simulink model "HDVPSG_DelayComp_NewRef_RealDrop_case1"  (R2019b)
settings: Solver=FixedStepDiscrete  StartTime=0.0  StopTime=28  FixedStep=UT.Ts_Veh  RelTol=1e-3
PostLoadFcn:
  | if any(exist('dsrtsu_mdlpostloadfcn', 'file') ~= 0), dsrtsu_mdlpostloadfcn('Execute', bdroot); end
InitFcn:
  | , if any(exist('dsmpb_private', 'file') ~= 0), dsmpb_private('dsmpb_mdlclblib', 'Init', bdroot); end,
values from neighbouring files (symbols this model uses):
  BETA_HDV_Leader = 50    [HDVPSG_DelayComp_NewRef_RealDrop_script_case1.m]
  BETA_PSG_Follower = 150    [HDVPSG_DelayComp_NewRef_RealDrop_script_case1.m]
  CtrlZone_Length = 250    [HDVPSG_DelayComp_NewRef_RealDrop_script_case1.m]
  DELTA_D_MIN = 5    [HDVPSG_DelayComp_NewRef_RealDrop_script_case1.m]
  DELTA_DR_MG_TCC = 15    [HDVPSG_DelayComp_NewRef_RealDrop_script_case1.m]
  HDV_AMAX = 1.3    [HDVPSG_DelayComp_NewRef_RealDrop_script_case1.m]
  HDV_AMIN = -2.5    [HDVPSG_DelayComp_NewRef_RealDrop_script_case1.m]
  HDV_first_v0 = 13    [HDVPSG_DelayComp_NewRef_RealDrop_script_case1.m]
  HDV_HighMu_D = 9    [HDVPSG_DelayComp_NewRef_RealDrop_script_case1.m]
  HDV_HighMu_I = 27    [HDVPSG_DelayComp_NewRef_RealDrop_script_case1.m]
  HDV_HighMu_P = 27    [HDVPSG_DelayComp_NewRef_RealDrop_script_case1.m]
  HDV_HighMu_TRFC = 0.7    [HDVPSG_DelayComp_NewRef_RealDrop_script_case1.m]
  HDV_last_v0 = 13    [HDVPSG_DelayComp_NewRef_RealDrop_script_case1.m]
  HDV_LowMu_D = 6    [HDVPSG_DelayComp_NewRef_RealDrop_script_case1.m]
  HDV_LowMu_I = 8    [HDVPSG_DelayComp_NewRef_RealDrop_script_case1.m]
  HDV_LowMu_P = 12    [HDVPSG_DelayComp_NewRef_RealDrop_script_case1.m]
  HDV_LowMu_TRFC = 0.6    [HDVPSG_DelayComp_NewRef_RealDrop_script_case1.m]
  Np_MPC = 20    [HDVPSG_DelayComp_NewRef_RealDrop_script_case1.m]
  PSG_AMAX = 3.2    [HDVPSG_DelayComp_NewRef_RealDrop_script_case1.m]
  PSG_AMIN = -6    [HDVPSG_DelayComp_NewRef_RealDrop_script_case1.m]
  PSG_end_v0 = 13    [HDVPSG_DelayComp_NewRef_RealDrop_script_case1.m]
  PSG_first_v0 = 13    [HDVPSG_DelayComp_NewRef_RealDrop_script_case1.m]
  PSG_HighMu_D = 15    [HDVPSG_DelayComp_NewRef_RealDrop_script_case1.m]
  PSG_HighMu_I = 125    [HDVPSG_DelayComp_NewRef_RealDrop_script_case1.m]
  PSG_HighMu_P = 75    [HDVPSG_DelayComp_NewRef_RealDrop_script_case1.m]
  PSG_HighMu_TRFC = 0.8    [HDVPSG_DelayComp_NewRef_RealDrop_script_case1.m]
  PSG_LowMu_D = 12    [HDVPSG_DelayComp_NewRef_RealDrop_script_case1.m]
  PSG_LowMu_I = 64    [HDVPSG_DelayComp_NewRef_RealDrop_script_case1.m]
  PSG_LowMu_P = 48    [HDVPSG_DelayComp_NewRef_RealDrop_script_case1.m]
  PSG_LowMu_TRFC = 0.7    [HDVPSG_DelayComp_NewRef_RealDrop_script_case1.m]
  PSG_middle_v0 = 13    [HDVPSG_DelayComp_NewRef_RealDrop_script_case1.m]
  Q_Leader = 1    [HDVPSG_DelayComp_NewRef_RealDrop_script_case1.m]
  Qd_dot_PSG_Follower = 2    [HDVPSG_DelayComp_NewRef_RealDrop_script_case1.m]
  Qd_PSG_Follower = 10    [HDVPSG_DelayComp_NewRef_RealDrop_script_case1.m]
  R_Leader = 20    [HDVPSG_DelayComp_NewRef_RealDrop_script_case1.m]
  R_PSG_Follower = 1    [HDVPSG_DelayComp_NewRef_RealDrop_script_case1.m]
  Recved_40_1 = Recved_Flag_Combined(47740,:)    [HDVPSG_DelayComp_NewRef_RealDrop_script_case1.m]
  Recved_40_2 = Recved_Flag_Combined(47780,:)    [HDVPSG_DelayComp_NewRef_RealDrop_script_case1.m]
  Recved_40_3 = Recved_Flag_Combined(49536,:)    [HDVPSG_DelayComp_NewRef_RealDrop_script_case1.m]
  Recved_40_4 = Recved_Flag_Combined(118106,:)    [HDVPSG_DelayComp_NewRef_RealDrop_script_case1.m]
  Rho_deltad_PSG_Follower = 1e3    (= 1000)    [HDVPSG_DelayComp_NewRef_RealDrop_script_case1.m]
  Rho_v_PSG_Follower = 1e3    (= 1000)    [HDVPSG_DelayComp_NewRef_RealDrop_script_case1.m]
  T_ADE = 0.01    [HDVPSG_DelayComp_NewRef_RealDrop_script_case1.m]
  V_MAX = 40    [HDVPSG_DelayComp_NewRef_RealDrop_script_case1.m]
  V_MIN = 0    [HDVPSG_DelayComp_NewRef_RealDrop_script_case1.m]
  VR_MG_TCC = 15    [HDVPSG_DelayComp_NewRef_RealDrop_script_case1.m]
undefined symbols (not defined in the file or in its folder): DiscIntNeverNeededParam, UT
libraries: simulink x46
(part 1 of 16)
PreSaveFcn:
  | , if any(exist('dsmpb_private', 'file') ~= 0), dsmpb_private('dsmpb_mdlclblib', 'PreSave', bdroot); end,
CloseFcn:
  | , if any(exist('dsmpb_private', 'file') ~= 0), dsmpb_private('dsmpb_mdlclblib', 'Close', bdroot); end,
settings Model: RTICANMMDATA=struct('GeneralSetupData',struct('modelroot',['C:\Program Files (x86)\Eclipse\Sumo\tools\contributed\traci4matlab\ZJ_Learn_Matlab4Traci\CVXGEN_ACM\acm-main\ACM_SUMO_ZJ\Simulink_With_Veh_Dynamics'],'generalsettings',struct('filesettings',struct('destfolder',struct('Name','RTICANMM_FILES','Check',1),'buildfolder',struct('Name','.','Check',1),'AbsDestfolder',struct('Name',['C:\Program Files (x86)\Eclipse\Sumo\tools\contributed\traci4matlab\ZJ_Learn_Matlab4Traci\CVXGEN_ACM\acm-main\ACM_SUMO_ZJ\Simulink_With_Veh_Dynamics\RTICANMM_FILES']),'AbsBuildfolder',struct('Name',['C:\Program Files (x86)\Eclipse\Sumo\tools\contributed\traci4matlab\ZJ_Learn_Matlab4Traci\CVXGEN_ACM\acm-main\ACM_SUMO_ZJ\Simulink_With_Veh_Dynamics']))),'options',struct('addpaths',1,'rmpaths',1,'addtrcexclusion',true,'cannavigator',struct('checkmonitoring',0),'show_usrtrc',0,'use_usrtrc',0),'advanced',struct('options',ones(1,100)),'MPSetup',{{}},'RTI',struct('Type','DSRT','Ver','4.2','Date','02-Nov-2019'),'modelname','HDVPSG_DelayComp_NewRef_RealDrop_case1','block','HDVPSG_DelayComp_NewRef_RealDrop_case1'))  DSRTSU_INTERNAL_RTIFPGA=150  Creator=znq  LastModifiedBy=znq
settings OptimizationCC: BlockReduction=off  ConditionallyExecuteInputs=off  OptimizeBlockIOStorage=off  BufferReuse=off  GlobalBufferReuse=off  ExpressionFolding=off  LocalBlockOutputs=off  OptimizeDataStoreBuffers=off  BusAssignmentInplaceUpdate=off
settings DebuggingCC: TasksWithSamePriorityMsg=none
settings HardwareCC: ProdBitPerPointer=32  ProdBitPerSizeT=32  ProdBitPerPtrDiffT=32  ProdLargestAtomicInteger=Integer  ProdWordSize=32  ProdHWDeviceType=Custom Processor->Custom
settings SFSimCC: MATLABDynamicMemAlloc=off
settings RTWCC: Description=dSPACE Run-Time Target (for VEOS on Windows and ConfigurationDesk)  SystemTargetFile=dsrt.tlc  GenCodeOnly=on  MakeCommand=make_dsrt  TemplateMakefile=dsrt_default_tmf  RTWVerbose=off
settings STFCustomTargetCC: TargetLangStandard=C99 (ISO)  ParMdlRefBuildCompliant=on  SystemTargetFile=dsrt.tlc
settings GRTTargetCC: CompOptLevelCompliant=off  ConcurrentExecutionCompliant=off  CombineOutputUpdateFcns=off  MatFileLogging=off  CPPClassGenCompliant=off  UseToolchainInfoCompliant=off

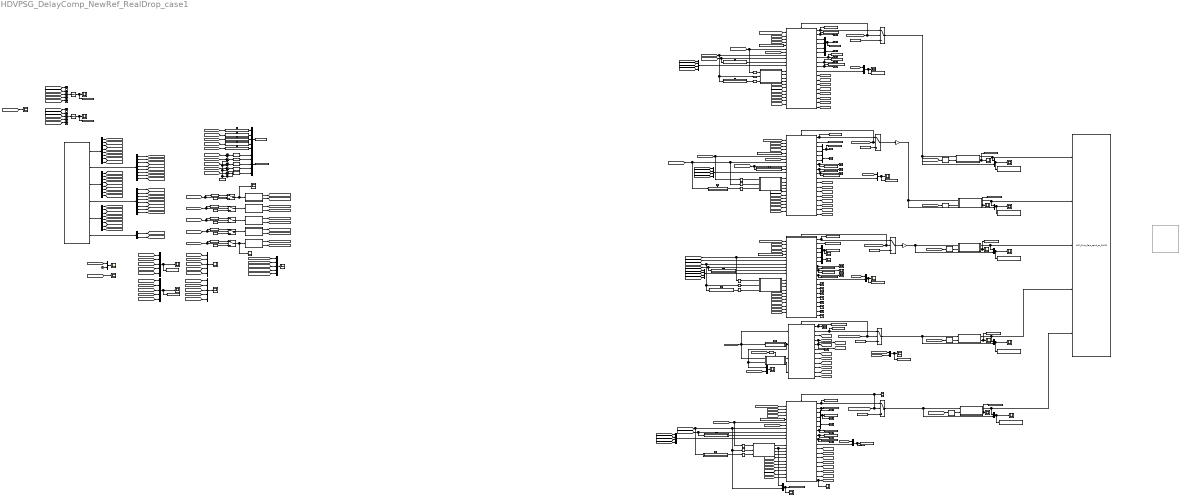
== system HDVPSG_DelayComp_NewRef_RealDrop_case1 ==
  note: We have reset the initial condition, such that FIFO is nautally set.
      | When PSG1 enters, it already has HDV2 inside the CTZ
      | You just say FIFO adopted, others refer to xxxx
  note: Here, we assume the a, v, d of a front car is send from that car, so, for instance, we do not need to calculate the a from its v, by ADE. If not, the control performance may be worsen.
  note: Vehicles Move Inside the Control Zone
  note: For all the merging participant, we assume their PDR are the same
      |
      | However, we cannot assume the package drops occur simutaneously between any two cars
      |
      | So, do not use the same Random Number generator seed
      |
      | Also, we assume the V2V package update rate for all the vehicles are the same
      |
      | Note the V2V package update rate != control rate = 0.01s
      |
      | V2V update slow, then a package drop will result in a longer unchanged V2V message (delay)
      |
      | A more realistic communication simulation may be done with NS3 (Omnet++)
  note: Comparison:
      | Opt / Opt + ULMPC
      | W/O self-prediction
      |
      | Other Seq / Other references refer to IV
      | XY Collision not needed anymore, as the new MP avoids lateral collsion
  ARE_First_Order_Derivative_[1,0,0]1 : Subsystem  TreatAsAtomicUnit=on
  ARE_First_Order_Derivative_[1,0,0]10 : Subsystem  TreatAsAtomicUnit=on
  ARE_First_Order_Derivative_[1,0,0]11 : Subsystem  TreatAsAtomicUnit=on
  ARE_First_Order_Derivative_[1,0,0]12 : Subsystem  TreatAsAtomicUnit=on
  ARE_First_Order_Derivative_[1,0,0]13 : Subsystem  TreatAsAtomicUnit=on
  ARE_First_Order_Derivative_[1,0,0]14 : Subsystem  TreatAsAtomicUnit=on
  ARE_First_Order_Derivative_[1,0,0]15 : Subsystem  TreatAsAtomicUnit=on
  ARE_First_Order_Derivative_[1,0,0]2 : Subsystem  TreatAsAtomicUnit=on
  ARE_First_Order_Derivative_[1,0,0]3 : Subsystem  TreatAsAtomicUnit=on
  ARE_First_Order_Derivative_[1,0,0]4 : Subsystem  TreatAsAtomicUnit=on
  ARE_First_Order_Derivative_[1,0,0]5 : Subsystem  TreatAsAtomicUnit=on
  ARE_First_Order_Derivative_[1,0,0]6 : Subsystem  TreatAsAtomicUnit=on
  ARE_First_Order_Derivative_[1,0,0]7 : Subsystem  TreatAsAtomicUnit=on
  ARE_First_Order_Derivative_[1,0,0]8 : Subsystem  TreatAsAtomicUnit=on
  ARE_First_Order_Derivative_[1,0,0]9 : Subsystem  TreatAsAtomicUnit=on
  Add1 : Sum  Inputs=5
  Add2 : Sum  Inputs=5
  Clock1 : Clock
  Compare To Constant1 : simulink/Logic and Bit Operations/Compare To Constant  relop===  const=1  OutDataTypeStr=boolean
  Constant1 : Constant  Value=2*DELTA_DR_MG_TCC/VR_MG_TCC
  Constant2 : Constant  Value=3*DELTA_DR_MG_TCC/VR_MG_TCC
  Constant3 : Constant  Value=4*DELTA_DR_MG_TCC/VR_MG_TCC
  Constant{42..45,50} (5 alike) : Constant  Value=10000
  Constant51 : Constant  Value=1*DELTA_DR_MG_TCC/VR_MG_TCC
  Constant52 : Constant  Value=HDV_first_v0
  Constant53 : Constant  Value=PSG_end_v0
  Constant54 : Constant  Value=PSG_middle_v0
  Constant55 : Constant  Value=PSG_first_v0
  Constant56 : Constant  Value=HDV_last_v0
  Demux{,2,5..7} (5 alike) : Demux  Outputs=8
  Demux8 : Demux  Outputs=2
  Discrete Derivative{,1..4} (5 alike) : simulink/Discrete/Discrete Derivative  gainval=1.0  ICPrevScaledInput=0.0  OutMin=[]  OutMax=[]  OutDataType=fixdt(1, 16)  OutScaling=2^-10  DoSatur=off
  Discrete-Time Integrator : DiscreteIntegrator  SampleTime=-1  ICPrevOutput=DiscIntNeverNeededParam  ICPrevScaledInput=DiscIntNeverNeededParam
  Discrete-Time Integrator1 : DiscreteIntegrator  SampleTime=-1  ICPrevOutput=DiscIntNeverNeededParam  ICPrevScaledInput=DiscIntNeverNeededParam
  Fcn{1..10} (10 alike) : Fcn  Expr=u-194
  Filter_Ts{1..13,15} (14 alike) : DiscretePulseGenerator  PulseType=Time based  Period=T_ADE*2  PulseWidth=50
  Gain : Gain
  Gain1 : Gain
  HDV2_control_withPDR_compen : Subsystem
  Level-2 MATLAB S-Function : M-S-Function  FunctionName=ACM_Five_Cars_send_to_SUMO
      mask Display: image('SUMO.png'); % Use "Edit Image" on toolstrip to change.
  Mux{,1..2,4..5,7..8,10..15,20..22,24..27,30} (21 alike) : Mux  Inputs=2
  Mux{16..19,28..29,32} (7 alike) : Mux  Inputs=5
  Mux{3,6,9,23} (4 alike) : Mux
  PSG1_control_withPDR_compen : Subsystem
  PSG2_control_withPDR_compen : Subsystem
  PSG3_control_withPDR_compen : Subsystem
  Rate Transition{,1..11} (12 alike) : RateTransition  OutPortSampleTime=V2V_SamplingPeriod
  Recv_5Cars_Data_From_SUMO : M-S-Function  FunctionName=ACM_Five_Cars_recv_from_SUMO
      mask Display: image('SUMO.png'); % Use "Edit Image" on toolstrip to change.
  Scope{,1..50,52..55} (55 alike) : Scope
  Subsystem1 : Subsystem
  Subsystem10 : Subsystem
  Subsystem11 : Subsystem
  Subsystem12 : Subsystem  Commented=on
  Subsystem13 : Subsystem
  Subsystem15 : Subsystem
  Subsystem2 : Subsystem
  Subsystem29 : Subsystem
  Subsystem3 : Subsystem
  Subsystem4 : Subsystem
  Subsystem5 : Subsystem
  Subsystem6 : Subsystem
  Subsystem7 : Subsystem
  Subsystem8 : Subsystem
  Subsystem9 : Subsystem
  Sum{,1..4} (5 alike) : Sum  Inputs=|++
  Switch{,4,7..9} (5 alike) : Switch  Criteria=u2 ~= 0
  Switch{3,5..6,10..11} (5 alike) : Switch  Criteria=u2 > Threshold
  Terminator{,1..7} (8 alike) : Terminator
  To Workspace : ToWorkspace  VariableName=PSG_First_vx_des_real  SaveFormat=Timeseries  SampleTime=-1
  To Workspace1 : ToWorkspace  VariableName=PSG_Middle_vx_des_real  SaveFormat=Timeseries  SampleTime=-1
  To Workspace10 : ToWorkspace  VariableName=deltav_cmd_PSG_End  SaveFormat=Timeseries  SampleTime=-1
  To Workspace11 : ToWorkspace  VariableName=deltav_cmd_HDV_First  SaveFormat=Timeseries  SampleTime=-1
  To Workspace12 : ToWorkspace  VariableName=v_cmd_HDV_First  SaveFormat=Timeseries  SampleTime=-1
  To Workspace13 : ToWorkspace  VariableName=deltav_cmd_HDV_Last  SaveFormat=Timeseries  SampleTime=-1
  To Workspace14 : ToWorkspace  VariableName=v_cmd_HDV_Last  SaveFormat=Timeseries  SampleTime=-1
  To Workspace15 : ToWorkspace  VariableName=v_vr_HDV_First  SaveFormat=Timeseries  SampleTime=-1
  To Workspace16 : ToWorkspace  VariableName=v_vr_PSG_First  SaveFormat=Timeseries  SampleTime=-1
  To Workspace17 : ToWorkspace  VariableName=v_vr_PSG_Middle  SaveFormat=Timeseries  SampleTime=-1
  To Workspace18 : ToWorkspace  VariableName=v_vr_PSG_End  SaveFormat=Timeseries  SampleTime=-1
  To Workspace19 : ToWorkspace  VariableName=v_vr_HDV_Last  SaveFormat=Timeseries  SampleTime=-1
  To Workspace2 : ToWorkspace  VariableName=PSG_End_vx_des_real  SaveFormat=Timeseries  SampleTime=-1
  To Workspace20 : ToWorkspace  VariableName=deltad_PSG_First  SaveFormat=Timeseries  SampleTime=-1
  To Workspace21 : ToWorkspace  VariableName=deltad_PSG_Middle  SaveFormat=Timeseries  SampleTime=-1
  To Workspace22 : ToWorkspace  VariableName=deltad_PSG_End  SaveFormat=Timeseries  SampleTime=-1
  To Workspace23 : ToWorkspace  VariableName=deltad_HDV_Last  SaveFormat=Timeseries  SampleTime=-1
  To Workspace24 : ToWorkspace  VariableName=Rhod_PSG_First  SaveFormat=Timeseries  SampleTime=-1
  To Workspace25 : ToWorkspace  VariableName=Absd_PSG_First  SaveFormat=Timeseries  SampleTime=-1
  To Workspace26 : ToWorkspace  VariableName=Rhod_PSG_Middle  SaveFormat=Timeseries  SampleTime=-1
  To Workspace27 : ToWorkspace  VariableName=Absd_PSG_Middle  SaveFormat=Timeseries  SampleTime=-1
  To Workspace28 : ToWorkspace  VariableName=Rhod_PSG_End  SaveFormat=Timeseries  SampleTime=-1
  To Workspace29 : ToWorkspace  VariableName=Absd_PSG_End  SaveFormat=Timeseries  SampleTime=-1
  To Workspace3 : ToWorkspace  VariableName=HDV_First_vx_des_real  SaveFormat=Timeseries  SampleTime=-1
  To Workspace30 : ToWorkspace  VariableName=Rhod_HDV_Last  SaveFormat=Timeseries  SampleTime=-1
  To Workspace31 : ToWorkspace  VariableName=Absd_HDV_Last  SaveFormat=Timeseries  SampleTime=-1
  To Workspace32 : ToWorkspace  VariableName=to_end_Summary  SaveFormat=Timeseries  SampleTime=-1
  To Workspace33 : ToWorkspace  VariableName=acc_Summary  SaveFormat=Timeseries  SampleTime=-1
  To Workspace34 : ToWorkspace  VariableName=ADE_Summary  SaveFormat=Timeseries  SampleTime=-1
  To Workspace35 : ToWorkspace  VariableName=DirectDiff_Summary  SaveFormat=Timeseries  SampleTime=-1
  To Workspace36 : ToWorkspace  VariableName=PSG_First_HighMu  SaveFormat=Timeseries  SampleTime=-1
  To Workspace37 : ToWorkspace  VariableName=PSG_Middle_HighMu  SaveFormat=Timeseries  SampleTime=-1
  To Workspace38 : ToWorkspace  VariableName=PSG_End_HighMu  SaveFormat=Timeseries  SampleTime=-1
  To Workspace39 : ToWorkspace  VariableName=HDV_First_HighMu  SaveFormat=Timeseries  SampleTime=-1
  To Workspace4 : ToWorkspace  VariableName=HDV_Last_vx_des_real  SaveFormat=Timeseries  SampleTime=-1
  To Workspace40 : ToWorkspace  VariableName=HDV_Last_HighMu  SaveFormat=Timeseries  SampleTime=-1
  To Workspace41 : ToWorkspace  VariableName=All_CO2  SaveFormat=Timeseries  SampleTime=-1
  To Workspace42 : ToWorkspace  VariableName=All_Fuel  SaveFormat=Timeseries  SampleTime=-1
  To Workspace43 : ToWorkspace  VariableName=Example_Package_Drop  SaveFormat=Timeseries  SampleTime=-1
  To Workspace44 : ToWorkspace  VariableName=deltad_agpdr_PSGEnd  SaveFormat=Timeseries  SampleTime=-1
  To Workspace45 : ToWorkspace  VariableName=deltad_agpdr_PSGMiddle  SaveFormat=Timeseries  SampleTime=-1
  To Workspace46 : ToWorkspace  VariableName=deltad_agpdr_PSGFirst  SaveFormat=Timeseries  SampleTime=-1
  To Workspace47 : ToWorkspace  VariableName=deltad_agpdr_HDV_Last  SaveFormat=Timeseries  SampleTime=-1
  To Workspace5 : ToWorkspace  VariableName=v_cmd_PSG_First  SaveFormat=Timeseries  SampleTime=-1
  To Workspace6 : ToWorkspace  VariableName=deltav_cmd_PSG_First  SaveFormat=Timeseries  SampleTime=-1
  To Workspace7 : ToWorkspace  VariableName=v_cmd_PSG_Middle  SaveFormat=Timeseries  SampleTime=-1
  To Workspace8 : ToWorkspace  VariableName=deltav_cmd_PSG_Middle  SaveFormat=Timeseries  SampleTime=-1
  To Workspace9 : ToWorkspace  VariableName=v_cmd_PSG_End  SaveFormat=Timeseries  SampleTime=-1
  Uniform Random Number : UniformRandomNumber  Minimum=-0.001  Maximum=0.001  Seed=122334  SampleTime=0.01
  leader_ulmpc_spd_ctrl : Subsystem
  wires:
  Recv_5Cars_Data_From_SUMO/1 -> Demux/1  "PSG_first"
  Recv_5Cars_Data_From_SUMO/2 -> Demux2/1  "PSG_middle"
  Recv_5Cars_Data_From_SUMO/3 -> Demux5/1  "PSG_end"
  Recv_5Cars_Data_From_SUMO/4 -> Demux6/1  "HDV_first"
  Recv_5Cars_Data_From_SUMO/5 -> Demux7/1  "HDV_last"
  Recv_5Cars_Data_From_SUMO/6 -> Demux8/1  "System"
  Demux/1 -> [x_PSG_first]
  Demux/2 -> [v_PSG_first]
  Demux/3 -> [a_PSG_first]
  Demux/4 -> [PSG_first_to_end]
  Demux/5 -> [co2_PSG_first]
  Demux/6 -> [fuel_PSG_first]
  Demux2/6 -> [fuel_PSG_middle]
  Demux2/5 -> [co2_PSG_middle]
  Demux2/4 -> [PSG_middle_to_end]
  Demux2/3 -> [a_PSG_middle]
  Demux2/2 -> [v_PSG_middle]
  Demux2/1 -> [x_PSG_middle]
  Demux5/1 -> [x_PSG_end]
  Demux5/2 -> [v_PSG_end]
  Demux5/3 -> [a_PSG_end]
  Demux5/4 -> [PSG_end_to_end]
  Demux5/5 -> [co2_PSG_end]
  Demux5/6 -> [fuel_PSG_end]
  Demux6/1 -> [x_HDV_first]
  Demux6/2 -> [v_HDV_first]
  Demux6/3 -> [a_HDV_first]
  Demux6/4 -> [HDV_first_to_end]
  Demux6/5 -> [co2_HDV_first]
  Demux6/6 -> [fuel_HDV_first]
  Demux7/1 -> [x_HDV_end]
  Demux7/2 -> [v_HDV_end]
  Demux7/3 -> [a_HDV_end]
  Demux7/4 -> [HDV_end_to_end]
  Demux7/5 -> [co2_HDV_end]
  Demux7/6 -> [fuel_HDV_end]
  Demux8/1 -> [SIM_STEP]
  Demux8/2 -> [Sumo_t]
  Clock1/1 -> Mux15/2
  Mux15/1 -> Scope34/1
  [Sumo_t] -> Mux15/1
  [SIM_STEP] -> Scope35/1
  [PSG_first_to_end] -> Mux16/1
  [PSG_middle_to_end] -> Mux16/2
  [PSG_end_to_end] -> Mux16/3
  [HDV_first_to_end] -> Mux16/4
  [HDV_end_to_end] -> Mux16/5
  Mux16/1 -> Scope36/1, To Workspace32/1
  Mux17/1 -> Scope37/1
  [x_PSG_first] -> Mux17/1
  [x_PSG_middle] -> Mux17/2
  [x_PSG_end] -> Mux17/3
  [x_HDV_first] -> Mux17/4
  [x_HDV_end] -> Mux17/5
  Mux18/1 -> Scope38/1
  [v_PSG_first] -> Mux18/1
  [v_PSG_middle] -> Mux18/2
  [v_PSG_end] -> Mux18/3
  [v_HDV_first] -> Mux18/4
  [v_HDV_end] -> Mux18/5
  Filter_Ts6/1 -> ARE_First_Order_Derivative_[1,0,0]6/Trigger
  Subsystem13/1(Ctrl_enabled) -> [HDV_first_Ctrl_enabled]
  Subsystem8/1(Ctrl_enabled) -> [HDV_end_Ctrl_enabled]
  Subsystem9/1(Ctrl_enabled) -> [PSG_first_Ctrl_enabled]
  Subsystem10/1(Ctrl_enabled) -> [PSG_middle_Ctrl_enabled]
  Subsystem11/1(Ctrl_enabled) -> [PSG_end_Ctrl_enabled]
  Mux14/1 -> To Workspace15/1, Scope33/1
  [HDV_first_Ctrl_enabled] -> leader_ulmpc_spd_ctrl/Enable, Switch5/2
  Constant52/1 -> Switch5/3
  Subsystem8/2(Ctrl_enable_Index) -> [HDV_end_Ctrlable_ind]
  Subsystem9/2(Ctrl_enable_Index) -> [PSG_first_Ctrlable_ind]
  Subsystem10/2(Ctrl_enable_Index) -> [PSG_middle_Ctrlable_ind]
  Subsystem11/2(Ctrl_enable_Index) -> [PSG_end_Ctrlable_ind]
  Subsystem13/2(Ctrl_enable_Index) -> [HDV_first_Ctrlable_ind]
  leader_ulmpc_spd_ctrl/2(v_cmd_opt) -> Switch5/1, To Workspace12/1  "v_cmd_HDV_first"
  leader_ulmpc_spd_ctrl/3(vr) -> [vr_HDV_first]
  ARE_First_Order_Derivative_[1,0,0]6/1(HDV_First_v_dot_hat) -> ARE_First_Order_Derivative_[1,0,0]3/2(HDV_First_a), Mux/1, leader_ulmpc_spd_ctrl/2(HDV_First_v_dot_hat)
  [v_HDV_first] -> ARE_First_Order_Derivative_[1,0,0]6/1(HDV_First_v), leader_ulmpc_spd_ctrl/1(HDV_First_v), ARE_First_Order_Derivative_[1,0,0]3/1(HDV_First_v)
  ARE_First_Order_Derivative_[1,0,0]3/1(HDV_First_v0_ctz) -> leader_ulmpc_spd_ctrl/3(spd_ini_ctzone)
  Compare To Constant1/1 -> ARE_First_Order_Derivative_[1,0,0]3/Enable
  [HDV_first_Ctrlable_ind] -> Compare To Constant1/1
  leader_ulmpc_spd_ctrl/1(delta_v_cmd_opt) -> To Workspace11/1, Scope8/1
  HDV2_control_withPDR_compen/1(v_cmd_opt) -> Switch6/1, To Workspace14/1  "v_cmd_HDV_first"
  Constant56/1 -> Switch6/3
  [HDV_end_Ctrl_enabled] -> Switch6/2, Scope52/1, HDV2_control_withPDR_compen/Enable
  Filter_Ts9/1 -> ARE_First_Order_Derivative_[1,0,0]10/Trigger
  leader_ulmpc_spd_ctrl/4(HDV1_t_all) -> [t_all_HDV1], [t_all_leader]
  [HDV_first_to_end] -> Fcn2/1, Switch/2
  Switch/1 -> Scope46/1, Subsystem13/1(dis_to_MP)
  Fcn2/1 -> Switch/1  "to_MP"
  Switch4/1 -> Subsystem8/1(dis_to_MP)
  Fcn3/1 -> Switch4/1  "to_MP"
  [HDV_end_to_end] -> Fcn3/1, Switch4/2
  [PSG_first_to_end] -> Fcn4/1, Switch7/2
  Fcn4/1 -> Switch7/1  "to_MP"
  Switch7/1 -> Subsystem9/1(dis_to_MP)
  Switch8/1 -> Subsystem10/1(dis_to_MP)
  Fcn5/1 -> Switch8/1  "to_MP"
  [PSG_middle_to_end] -> Fcn5/1, Switch8/2
  [PSG_end_to_end] -> Fcn6/1, Switch9/2
  Fcn6/1 -> Switch9/1  "to_MP"
  Switch9/1 -> Scope55/1, Subsystem11/1(dis_to_MP)
  Constant42/1 -> Switch/3
  Constant43/1 -> Switch4/3
  Constant44/1 -> Switch7/3
  Constant45/1 -> Switch8/3
  Constant50/1 -> Switch9/3
  [HDV_end_Ctrlable_ind] -> HDV2_control_withPDR_compen/1(Ego_CtrL_enabled_Index)
  [v_HDV_end] -> ARE_First_Order_Derivative_[1,0,0]7/1(HDV_last_v), HDV2_control_withPDR_compen/9(v_Ego)
  HDV2_control_withPDR_compen/3(delta_dr) -> Mux21/1
  HDV2_control_withPDR_compen/4(delta_d) -> Mux21/2
  HDV2_control_withPDR_compen/6(delta_d_dot) -> Mux22/2
  Mux21/1 -> Scope1/1, To Workspace23/1
  Mux22/1 -> Scope3/1
  [t_all_leader] -> HDV2_control_withPDR_compen/2(t_all_leader)
  Constant51/1 -> HDV2_control_withPDR_compen/5(Time_headway)
  [HDV_end_to_end] -> HDV2_control_withPDR_compen/7(Ego_to_end)
  ARE_First_Order_Derivative_[1,0,0]7/1(HDV_last_v_dot_hat) -> HDV2_control_withPDR_compen/10(a_Ego)
  Constant53/1 -> Switch10/3
  [PSG_middle_Ctrl_enabled] -> PSG2_control_withPDR_compen/Enable, Switch3/2
  Constant54/1 -> Switch3/3
  Constant55/1 -> Switch11/3
  [PSG_first_Ctrl_enabled] -> Switch11/2, PSG1_control_withPDR_compen/Enable
  Demux/7 -> [X_PSG_first]
  Demux5/7 -> [X_PSG_end]
  Demux7/7 -> [X_HDV_end]
  Demux6/7 -> [X_HDV_first]
  Demux2/7 -> [X_PSG_middle]
  Filter_Ts3/1 -> ARE_First_Order_Derivative_[1,0,0]7/Trigger
  Demux2/8 -> [Y_PSG_middle]
  Demux5/8 -> [Y_PSG_end]
  Demux6/8 -> [Y_HDV_first]
  Demux7/8 -> [Y_HDV_end]
  Demux/8 -> [Y_PSG_first]
  [X_HDV_end] -> Mux23/1
  [Y_HDV_end] -> Mux23/2
  [X_HDV_first] -> Mux23/3
  [Y_HDV_first] -> Mux23/4
  HDV2_control_withPDR_compen/7(Rho_d_adapt) -> Scope4/1, To Workspace30/1
  HDV2_control_withPDR_compen/8(AbsDis_ego_front) -> Scope2/1, To Workspace31/1
  HDV2_control_withPDR_compen/2(deltav_cmd_opt) -> Scope5/1, To Workspace13/1
  Filter_Ts1/1 -> ARE_First_Order_Derivative_[1,0,0]2/Trigger
  Mux2/1 -> Scope7/1
  Mux1/1 -> Scope9/1, To Workspace20/1
  [v_PSG_first] -> ARE_First_Order_Derivative_[1,0,0]2/1(PSG_first_v), PSG1_control_withPDR_compen/9(v_Ego)
  Filter_Ts2/1 -> ARE_First_Order_Derivative_[1,0,0]1/Trigger
  [X_HDV_end] -> Mux3/3
  [Y_HDV_end] -> Mux3/4
  [X_PSG_first] -> Mux3/1
  [Y_PSG_first] -> Mux3/2
  Filter_Ts5/1 -> ARE_First_Order_Derivative_[1,0,0]4/Trigger
  [v_PSG_middle] -> ARE_First_Order_Derivative_[1,0,0]5/1(PSG_middle_v), PSG2_control_withPDR_compen/9(v_Ego)
  Mux4/1 -> To Workspace21/1, Scope12/1
  Mux5/1 -> Scope16/1
  Filter_Ts4/1 -> ARE_First_Order_Derivative_[1,0,0]5/Trigger
  PSG2_control_withPDR_compen/7(Rho_d_adapt) -> To Workspace26/1, Scope14/1
  PSG2_control_withPDR_compen/8(AbsDis_ego_front) -> Scope15/1, To Workspace27/1
  [X_PSG_first] -> Mux6/3
  [Y_PSG_first] -> Mux6/4
  [X_PSG_middle] -> Mux6/1
  [Y_PSG_middle] -> Mux6/2
  PSG3_control_withPDR_compen/8(AbsDis_ego_front) -> Scope20/1, To Workspace29/1
  PSG3_control_withPDR_compen/7(Rho_d_adapt) -> Scope19/1, To Workspace28/1
  Filter_Ts7/1 -> ARE_First_Order_Derivative_[1,0,0]9/Trigger
  Mux8/1 -> Scope21/1
  Mux7/1 -> Scope17/1, To Workspace22/1
  PSG3_control_withPDR_compen/6(delta_d_dot) -> Mux8/2
  PSG3_control_withPDR_compen/5(delta_dr_dot) -> Mux8/1
  [v_PSG_end] -> PSG3_control_withPDR_compen/9(v_Ego), ARE_First_Order_Derivative_[1,0,0]9/1(PSG_end_v)
  Filter_Ts8/1 -> ARE_First_Order_Derivative_[1,0,0]8/Trigger
  [PSG_end_Ctrl_enabled] -> PSG3_control_withPDR_compen/Enable, Switch10/2
  [Y_PSG_middle] -> Mux9/4
  [X_PSG_middle] -> Mux9/3
  [X_PSG_end] -> Mux9/1
  [Y_PSG_end] -> Mux9/2
  Mux24/1 -> To Workspace16/1, Scope26/1
  [vr_HDV_first] -> Mux14/2
  [v_HDV_first] -> Mux14/1
  [v_PSG_first] -> Mux24/1
  PSG1_control_withPDR_compen/10(opt_spd) -> Mux24/2
  [v_PSG_middle] -> Mux25/1
  Mux25/1 -> To Workspace17/1, Scope27/1
  Mux26/1 -> Scope28/1, To Workspace18/1
  [v_PSG_end] -> Mux26/1
  HDV2_control_withPDR_compen/10(opt_spd) -> Mux27/2
  [v_HDV_end] -> Mux27/1
  Mux27/1 -> Scope29/1, To Workspace19/1
  HDV2_control_withPDR_compen/5(delta_dr_dot) -> Mux22/1
  Mux19/1 -> To Workspace33/1, Scope30/1
  [a_PSG_end] -> Mux19/3
  [a_PSG_middle] -> Mux19/2
  [a_PSG_first] -> Mux19/1
  [a_HDV_end] -> Mux19/5
  [a_HDV_first] -> Mux19/4
  Filter_Ts10/1 -> ARE_First_Order_Derivative_[1,0,0]11/Trigger
  [v_HDV_end] -> ARE_First_Order_Derivative_[1,0,0]11/1(HDV_last_v)
  Filter_Ts11/1 -> ARE_First_Order_Derivative_[1,0,0]12/Trigger
  [v_PSG_first] -> ARE_First_Order_Derivative_[1,0,0]12/1(PSG_first_v)
  Filter_Ts12/1 -> ARE_First_Order_Derivative_[1,0,0]13/Trigger
  [v_PSG_middle] -> ARE_First_Order_Derivative_[1,0,0]13/1(PSG_middle_v)
  Filter_Ts13/1 -> ARE_First_Order_Derivative_[1,0,0]14/Trigger
  [v_HDV_first] -> ARE_First_Order_Derivative_[1,0,0]14/1(HDV_first_v)
  Filter_Ts15/1 -> ARE_First_Order_Derivative_[1,0,0]15/Trigger
  [v_PSG_end] -> ARE_First_Order_Derivative_[1,0,0]15/1(PSG_end_v)
  ARE_First_Order_Derivative_[1,0,0]12/1(PSG_first_v_dot_hat) -> Mux28/1
  ARE_First_Order_Derivative_[1,0,0]13/1(PSG_middle_v_dot_hat) -> Mux28/2
  ARE_First_Order_Derivative_[1,0,0]15/1(PSG_end_v_dot_hat) -> Mux28/3
  ARE_First_Order_Derivative_[1,0,0]14/1(HDV_first_v_dot_hat) -> Mux28/4
  ARE_First_Order_Derivative_[1,0,0]11/1(HDV_last_v_dot_hat) -> Mux28/5
  Mux28/1 -> To Workspace34/1
  Mux29/1 -> To Workspace35/1
  Discrete Derivative/1 -> Mux29/1
  Discrete Derivative1/1 -> Mux29/2
  Discrete Derivative2/1 -> Mux29/3
  Discrete Derivative3/1 -> Mux29/4
  Discrete Derivative4/1 -> Mux29/5
  Sum/1 -> Discrete Derivative/1
  [v_PSG_first] -> Sum/1
  Sum1/1 -> Discrete Derivative1/1
  Sum2/1 -> Discrete Derivative2/1
  [v_PSG_end] -> Sum2/1
  [v_PSG_middle] -> Sum1/1
  Sum3/1 -> Discrete Derivative3/1
  [v_HDV_first] -> Sum3/1
  Sum4/1 -> Discrete Derivative4/1
  [v_HDV_end] -> Sum4/1
  Uniform Random Number/1 -> Sum/2, Sum1/2, Sum2/2, Sum3/2, Sum4/2
  leader_ulmpc_spd_ctrl/5(HDV1_Run_t) -> [t_hasrun_HDV1], [leader_ran_t]
  [leader_ran_t] -> HDV2_control_withPDR_compen/3(t_leader_has_run)
  Fcn10/1 -> Subsystem3/2(Dist_to_MP)  "to_MP"
  Subsystem3/1(vx_HDV_end) -> Mux20/1, Level-2 MATLAB S-Function/5
  [HDV_first_to_end] -> Fcn9/1
  Mux10/1 -> To Workspace3/1, Scope25/1
  Switch5/1 -> Mux10/2, Subsystem6/1(vxr_HDV_first)
  Switch6/1 -> Mux20/2, Subsystem3/1(vxr_HDV_end)
  Subsystem2/1(vx_PSG_end) -> Mux11/1, Level-2 MATLAB S-Function/3
  Fcn8/1 -> Subsystem2/2(Dist_to_MP)  "to_MP"
  [HDV_end_to_end] -> Fcn10/1
  Subsystem1/1(vx_PSG_middle) -> Mux12/1, Level-2 MATLAB S-Function/2
  Subsystem2/2(HighMu) -> To Workspace38/1, Scope11/1
  Fcn7/1 -> Subsystem1/2(Dist_to_MP)  "to_MP"
  Subsystem6/1(vx_HDV_first) -> Mux10/1, Level-2 MATLAB S-Function/4
  Mux20/1 -> To Workspace4/1, Scope41/1
  [PSG_middle_to_end] -> Fcn7/1
  Switch11/1 -> Mux13/2, Subsystem29/1(vxr_PSG_first)
  Mux11/1 -> To Workspace2/1, Scope32/1
  [PSG_first_to_end] -> Fcn1/1
  Switch3/1 -> Gain/1
  [PSG_end_to_end] -> Fcn8/1
  Mux12/1 -> To Workspace1/1, Scope39/1
  Subsystem29/1(vx_PSG_first) -> Mux13/1, Level-2 MATLAB S-Function/1
  Switch10/1 -> Gain1/1
  Subsystem29/2(HighMu) -> To Workspace36/1, Scope24/1
  Subsystem1/2(HighMu) -> To Workspace37/1, Scope42/1
  Subsystem6/2(HighMu) -> To Workspace39/1, Scope22/1
  Fcn9/1 -> Subsystem6/2(Dist_to_MP)  "to_MP"
  Mux13/1 -> To Workspace/1, Scope40/1
  Subsystem3/2(HighMu) -> To Workspace40/1, Scope23/1
  Fcn1/1 -> Subsystem29/2(Dist_to_MP)  "to_MP"
  [v_HDV_first] -> Mux30/2, Rate Transition1/1, HDV2_control_withPDR_compen/8(v_Front), ARE_First_Order_Derivative_[1,0,0]10/1(HDV_first_v)
  ARE_First_Order_Derivative_[1,0,0]10/1(HDV_first_v_dot_hat) -> Rate Transition/1
  [HDV_first_to_end] -> Rate Transition2/1, HDV2_control_withPDR_compen/6(Front_to_end)
  Subsystem15/1(Front_to_end_PDR) -> HDV2_control_withPDR_compen/13(Front_to_end_PDR)
  Subsystem15/2(v_Front_PDR) -> Mux30/1, HDV2_control_withPDR_compen/14(v_Front_PDR)
  Subsystem15/3(a_Front_PDR) -> HDV2_control_withPDR_compen/15(a_Front_PDR)
  [v_HDV_end] -> PSG1_control_withPDR_compen/8(v_Front), Rate Transition10/1, ARE_First_Order_Derivative_[1,0,0]1/1(HDV_last_v)
  [HDV_end_to_end] -> PSG1_control_withPDR_compen/6(Front_to_end), Rate Transition9/1
  ARE_First_Order_Derivative_[1,0,0]1/1(HDV_last_v_dot_hat) -> Rate Transition11/1
  ARE_First_Order_Derivative_[1,0,0]4/1(PSG_first_v_dot_hat) -> Rate Transition5/1
  [PSG_first_to_end] -> PSG2_control_withPDR_compen/6(Front_to_end), Rate Transition3/1
  [v_PSG_first] -> PSG2_control_withPDR_compen/8(v_Front), Rate Transition4/1, ARE_First_Order_Derivative_[1,0,0]4/1(PSG_first_v)
  [v_PSG_middle] -> Rate Transition7/1, ARE_First_Order_Derivative_[1,0,0]8/1(PSG_middle_v), PSG3_control_withPDR_compen/8(v_Front)
  [PSG_middle_to_end] -> PSG3_control_withPDR_compen/6(Front_to_end), Rate Transition8/1
  ARE_First_Order_Derivative_[1,0,0]8/1(PSG_middle_v_dot_hat) -> Rate Transition6/1
  [co2_HDV_end] -> Add1/2
  [co2_HDV_first] -> Add1/1
  [co2_PSG_middle] -> Add1/4
  [co2_PSG_first] -> Add1/3
  [co2_PSG_end] -> Add1/5
  [fuel_PSG_first] -> Add2/3
  [fuel_HDV_end] -> Add2/2
  [fuel_HDV_first] -> Add2/1
  [fuel_PSG_middle] -> Add2/4
  [fuel_PSG_end] -> Add2/5
  Mux30/1 -> Scope44/1, To Workspace43/1
  Add1/1 -> Discrete-Time Integrator/1
  Discrete-Time Integrator/1 -> To Workspace41/1, Scope/1
  Add2/1 -> Discrete-Time Integrator1/1
  Discrete-Time Integrator1/1 -> To Workspace42/1, Scope43/1
  Rate Transition8/1 -> Subsystem7/1(Front_to_end)
  Rate Transition7/1 -> Subsystem7/2(v_Front)
  Rate Transition6/1 -> Subsystem7/3(a_Front)
  Rate Transition3/1 -> Subsystem4/1(Front_to_end)
  Rate Transition4/1 -> Subsystem4/2(v_Front)
  Rate Transition5/1 -> Subsystem4/3(a_Front)
  Rate Transition9/1 -> Subsystem5/1(Front_to_end)
  Rate Transition10/1 -> Subsystem5/2(v_Front)
  Rate Transition11/1 -> Subsystem5/3(a_Front)
  [fuel_HDV_end] -> Scope45/1
  PSG3_control_withPDR_compen/1(v_cmd_opt) -> Switch10/1, To Workspace9/1
  PSG3_control_withPDR_compen/2(deltav_cmd_opt) -> To Workspace10/1
  PSG3_control_withPDR_compen/3(delta_dr) -> Mux7/1
  PSG3_control_withPDR_compen/4(delta_d) -> Mux7/2
  PSG3_control_withPDR_compen/9(delta_d_against_PDR) -> Scope18/1, To Workspace44/1
  PSG2_control_withPDR_compen/9(delta_d_against_PDR) -> Scope13/1, To Workspace45/1
  PSG2_control_withPDR_compen/1(v_cmd_opt) -> To Workspace7/1, Switch3/1
  PSG2_control_withPDR_compen/2(deltav_cmd_opt) -> To Workspace8/1
  PSG2_control_withPDR_compen/4(delta_d) -> Mux4/2
  PSG2_control_withPDR_compen/3(delta_dr) -> Mux4/1
  PSG2_control_withPDR_compen/5(delta_dr_dot) -> Mux5/1
  PSG2_control_withPDR_compen/6(delta_d_dot) -> Mux5/2
  [PSG_first_Ctrlable_ind] -> PSG1_control_withPDR_compen/1(Ego_CtrL_enabled_Index)
  [t_all_leader] -> PSG1_control_withPDR_compen/2(t_all_leader)
  [leader_ran_t] -> PSG1_control_withPDR_compen/3(t_leader_has_run)
  Constant1/1 -> PSG1_control_withPDR_compen/5(Time_headway)
  PSG1_control_withPDR_compen/1(v_cmd_opt) -> Switch11/1, To Workspace5/1
  PSG1_control_withPDR_compen/2(deltav_cmd_opt) -> To Workspace6/1, Scope10/1
  PSG1_control_withPDR_compen/8(AbsDis_ego_front) -> Scope31/1, To Workspace25/1
  PSG1_control_withPDR_compen/7(Rho_d_adapt) -> Scope6/1, To Workspace24/1
  PSG1_control_withPDR_compen/5(delta_dr_dot) -> Mux2/1
  PSG1_control_withPDR_compen/6(delta_d_dot) -> Mux2/2
  PSG1_control_withPDR_compen/3(delta_dr) -> Mux1/1
  PSG1_control_withPDR_compen/4(delta_d) -> Mux1/2
  PSG1_control_withPDR_compen/9(delta_d_against_PDR) -> Scope47/1, To Workspace46/1
  Mux23/1 -> HDV2_control_withPDR_compen/11(XY_ego_front)
  HDV2_control_withPDR_compen/9(delta_d_against_PDR) -> To Workspace47/1, Scope48/1
  Subsystem15/4(Recved) -> HDV2_control_withPDR_compen/16(Recved)
  ARE_First_Order_Derivative_[1,0,0]3/2(HDV_First_a0_ctz) -> leader_ulmpc_spd_ctrl/4(acc_ini_ctzone)
  Mux/1 -> Scope49/1
  [a_HDV_first] -> Mux/2
  leader_ulmpc_spd_ctrl/6(opt_dist2MP) -> Scope50/1
  [t_all_HDV1] -> HDV2_control_withPDR_compen/23(T_all_to_MP_pre)
  [t_hasrun_HDV1] -> HDV2_control_withPDR_compen/4(t_PRE_has_run)
  leader_ulmpc_spd_ctrl/7(alpha_HDV1) -> [alpha_HDV1]
  leader_ulmpc_spd_ctrl/8(beta_HDV1) -> [beta_HDV1]
  leader_ulmpc_spd_ctrl/9(c1_HDV1) -> [c1_HDV1]
  leader_ulmpc_spd_ctrl/10(c2_HDV1) -> [c2_HDV1]
  leader_ulmpc_spd_ctrl/11(c3_HDV1) -> [c3_HDV1]
  leader_ulmpc_spd_ctrl/12(c4_HDV1) -> [c4_HDV1]
  [alpha_HDV1] -> HDV2_control_withPDR_compen/17(alpha_pre)
  [beta_HDV1] -> HDV2_control_withPDR_compen/18(beta_pre)
  [c1_HDV1] -> HDV2_control_withPDR_compen/19(c_1_pre)
  [c2_HDV1] -> HDV2_control_withPDR_compen/20(c_2_pre)
  [c3_HDV1] -> HDV2_control_withPDR_compen/21(c_3_pre)
  [c4_HDV1] -> HDV2_control_withPDR_compen/22(c_4_pre)
  HDV2_control_withPDR_compen/11(alpha_HDV2) -> [alpha_HDV2]
  HDV2_control_withPDR_compen/12(beta_HDV2) -> [beta_HDV2]
  HDV2_control_withPDR_compen/13(c1_HDV2) -> [c1_HDV2]
  HDV2_control_withPDR_compen/14(c2_HDV2) -> [c2_HDV2]
  HDV2_control_withPDR_compen/15(c3_HDV2) -> [c3_HDV2]
  HDV2_control_withPDR_compen/16(c4_HDV2) -> [c4_HDV2]
  HDV2_control_withPDR_compen/17(Tall_to_MP_HDV2) -> [t_all_HDV2]
  HDV2_control_withPDR_compen/18(t_hasrun_HDV2) -> Scope53/1, [t_hasrun_HDV2]
  [c1_HDV2] -> PSG1_control_withPDR_compen/19(c_1_pre)
  [c2_HDV2] -> PSG1_control_withPDR_compen/20(c_2_pre)
  [c3_HDV2] -> PSG1_control_withPDR_compen/21(c_3_pre)
  [c4_HDV2] -> PSG1_control_withPDR_compen/22(c_4_pre)
  [t_all_HDV2] -> PSG1_control_withPDR_compen/23(T_all_to_MP_pre)
  [beta_HDV2] -> PSG1_control_withPDR_compen/18(beta_pre)
  [alpha_HDV2] -> PSG1_control_withPDR_compen/17(alpha_pre)
  [t_hasrun_HDV2] -> PSG1_control_withPDR_compen/4(t_PRE_has_run)
  Subsystem5/4(Recved) -> PSG1_control_withPDR_compen/16(Recved)
  Subsystem5/3(a_Front_PDR) -> PSG1_control_withPDR_compen/15(a_Front_PDR)
  Subsystem5/2(v_Front_PDR) -> PSG1_control_withPDR_compen/14(v_Front_PDR)
  Subsystem5/1(Front_to_end_PDR) -> PSG1_control_withPDR_compen/13(Front_to_end_PDR)
  [PSG_first_to_end] -> PSG1_control_withPDR_compen/7(Ego_to_end)
  ARE_First_Order_Derivative_[1,0,0]2/1(PSG_first_v_dot_hat) -> PSG1_control_withPDR_compen/10(a_Ego)
  Mux3/1 -> PSG1_control_withPDR_compen/11(XY_ego_front)
  PSG1_control_withPDR_compen/11(alpha_PSG1) -> [alpha_PSG1]
  PSG1_control_withPDR_compen/12(beta_PSG1) -> [beta_PSG1]
  PSG1_control_withPDR_compen/13(c1_PSG1) -> [c1_PSG1]
  PSG1_control_withPDR_compen/14(c2_PSG1) -> [c2_PSG1]
  PSG1_control_withPDR_compen/15(c3_PSG1) -> [c3_PSG1]
  PSG1_control_withPDR_compen/16(c4_PSG1) -> [c4_PSG1]
  PSG1_control_withPDR_compen/17(Tall_to_MP_PSG1) -> [t_all_PSG1]
  PSG1_control_withPDR_compen/18(t_hasrun_PSG1) -> [t_hasrun_PSG1]
  Gain/1 -> Subsystem1/1(vxr_PSG_middle), Mux12/2
  Gain1/1 -> Mux11/2, Subsystem2/1(vxr_PSG_end)
  [PSG_end_Ctrlable_ind] -> Mux32/5
  [PSG_middle_Ctrlable_ind] -> Mux32/4
  [PSG_first_Ctrlable_ind] -> Mux32/3
  [HDV_end_Ctrlable_ind] -> Mux32/2
  [HDV_first_Ctrlable_ind] -> Mux32/1
  Mux32/1 -> Scope54/1
  [c1_PSG1] -> PSG2_control_withPDR_compen/19(c_1_pre)
  [c2_PSG1] -> PSG2_control_withPDR_compen/20(c_2_pre)
  [c3_PSG1] -> PSG2_control_withPDR_compen/21(c_3_pre)
  [c4_PSG1] -> PSG2_control_withPDR_compen/22(c_4_pre)
  [t_all_PSG1] -> PSG2_control_withPDR_compen/23(T_all_to_MP_pre)
  [beta_PSG1] -> PSG2_control_withPDR_compen/18(beta_pre)
  [alpha_PSG1] -> PSG2_control_withPDR_compen/17(alpha_pre)
  [t_hasrun_PSG1] -> PSG2_control_withPDR_compen/4(t_PRE_has_run)
  [PSG_middle_Ctrlable_ind] -> PSG2_control_withPDR_compen/1(Ego_CtrL_enabled_Index)
  [t_all_leader] -> PSG2_control_withPDR_compen/2(t_all_leader)
  [leader_ran_t] -> PSG2_control_withPDR_compen/3(t_leader_has_run)
  Constant2/1 -> PSG2_control_withPDR_compen/5(Time_headway)
  [PSG_middle_to_end] -> PSG2_control_withPDR_compen/7(Ego_to_end)
  ARE_First_Order_Derivative_[1,0,0]5/1(PSG_middle_v_dot_hat) -> PSG2_control_withPDR_compen/10(a_Ego)
  Subsystem4/1(Front_to_end_PDR) -> PSG2_control_withPDR_compen/13(Front_to_end_PDR)
  Subsystem4/2(v_Front_PDR) -> PSG2_control_withPDR_compen/14(v_Front_PDR)
  Subsystem4/3(a_Front_PDR) -> PSG2_control_withPDR_compen/15(a_Front_PDR)
  Subsystem4/4(Recved) -> PSG2_control_withPDR_compen/16(Recved)
  Mux6/1 -> PSG2_control_withPDR_compen/11(XY_ego_front)
  PSG2_control_withPDR_compen/10(opt_spd) -> Mux25/2
  PSG2_control_withPDR_compen/11(alpha_PSG2) -> [alpha_PSG2]
  PSG2_control_withPDR_compen/12(beta_PSG2) -> [beta_PSG2]
  PSG2_control_withPDR_compen/13(c1_PSG2) -> [c1_PSG2]
  PSG2_control_withPDR_compen/14(c2_PSG2) -> [c2_PSG2]
  PSG2_control_withPDR_compen/15(c3_PSG2) -> [c3_PSG2]
  PSG2_control_withPDR_compen/16(c4_PSG2) -> [c4_PSG2]
  PSG2_control_withPDR_compen/17(Tall_to_MP_PSG2) -> [t_all_PSG2]
  PSG2_control_withPDR_compen/18(t_hasrun_PSG2) -> [t_hasrun_PSG2]
  [alpha_PSG2] -> PSG3_control_withPDR_compen/17(alpha_pre)
  [beta_PSG2] -> PSG3_control_withPDR_compen/18(beta_pre)
  [c1_PSG2] -> PSG3_control_withPDR_compen/19(c_1_pre)
  [c2_PSG2] -> PSG3_control_withPDR_compen/20(c_2_pre)
  [c3_PSG2] -> PSG3_control_withPDR_compen/21(c_3_pre)
  [c4_PSG2] -> PSG3_control_withPDR_compen/22(c_4_pre)
  [t_all_PSG2] -> PSG3_control_withPDR_compen/23(T_all_to_MP_pre)
  [t_hasrun_PSG2] -> PSG3_control_withPDR_compen/4(t_PRE_has_run)
  [PSG_end_Ctrlable_ind] -> PSG3_control_withPDR_compen/1(Ego_CtrL_enabled_Index)
  [t_all_leader] -> PSG3_control_withPDR_compen/2(t_all_leader)
  [leader_ran_t] -> PSG3_control_withPDR_compen/3(t_leader_has_run)
  Constant3/1 -> PSG3_control_withPDR_compen/5(Time_headway)
  Subsystem7/4(Recved) -> PSG3_control_withPDR_compen/16(Recved)
  Subsystem7/3(a_Front_PDR) -> PSG3_control_withPDR_compen/15(a_Front_PDR)
  Subsystem7/2(v_Front_PDR) -> PSG3_control_withPDR_compen/14(v_Front_PDR)
  Subsystem7/1(Front_to_end_PDR) -> PSG3_control_withPDR_compen/13(Front_to_end_PDR)
  [PSG_end_to_end] -> PSG3_control_withPDR_compen/7(Ego_to_end)
  ARE_First_Order_Derivative_[1,0,0]9/1(PSG_end_v_dot_hat) -> PSG3_control_withPDR_compen/10(a_Ego)
  Mux9/1 -> PSG3_control_withPDR_compen/11(XY_ego_front)
  PSG3_control_withPDR_compen/11(alpha_PSG3) -> Terminator/1
  PSG3_control_withPDR_compen/12(beta_PSG3) -> Terminator1/1
  PSG3_control_withPDR_compen/13(c1_PSG3) -> Terminator2/1
  PSG3_control_withPDR_compen/14(c2_PSG3) -> Terminator3/1
  PSG3_control_withPDR_compen/15(c3_PSG3) -> Terminator4/1
  PSG3_control_withPDR_compen/16(c4_PSG3) -> Terminator5/1
  PSG3_control_withPDR_compen/17(Tall_to_MP_PSG3) -> Terminator6/1
  PSG3_control_withPDR_compen/18(t_hasrun_PSG3) -> Terminator7/1
  PSG3_control_withPDR_compen/10(opt_spd) -> Mux26/2
  Rate Transition/1 -> Subsystem15/3(a_Front)
  Rate Transition1/1 -> Subsystem15/2(v_Front)
  Rate Transition2/1 -> Subsystem15/1(Front_to_end)

== system HDVPSG_DelayComp_NewRef_RealDrop_case1/ARE_First_Order_Derivative_[1,0,0]1 ==
  HDV_last_v : Inport
  Trigger : TriggerPort  TriggerType=either  VariantControl=Variant  ZeroCross=off  PortDimensions=1
  Constant : Constant  Value=T_ADE
  Constant52 : Constant  Value=HDV_last_v0
  MATLAB Function : MATLAB Function  TreatAsAtomicUnit=on
  HDV_last_v_dot_hat : Outport  VectorParamsAs1DForOutWhenUnconnected=off
  wires:
  Constant52/1 -> MATLAB Function/3(u_init)
  HDV_last_v/1 -> MATLAB Function/1(U)
  MATLAB Function/1(Dot_U) -> HDV_last_v_dot_hat/1
  Constant/1 -> MATLAB Function/2(Ts)

== system HDVPSG_DelayComp_NewRef_RealDrop_case1/ARE_First_Order_Derivative_[1,0,0]10 ==
  HDV_first_v : Inport
  Trigger : TriggerPort  TriggerType=either  VariantControl=Variant  ZeroCross=off  PortDimensions=1
  Constant : Constant  Value=T_ADE
  Constant52 : Constant  Value=HDV_first_v0
  MATLAB Function : MATLAB Function  TreatAsAtomicUnit=on
  HDV_first_v_dot_hat : Outport  VectorParamsAs1DForOutWhenUnconnected=off
  wires:
  Constant/1 -> MATLAB Function/2(Ts)
  MATLAB Function/1(Dot_U) -> HDV_first_v_dot_hat/1
  HDV_first_v/1 -> MATLAB Function/1(U)
  Constant52/1 -> MATLAB Function/3(u_init)

== system HDVPSG_DelayComp_NewRef_RealDrop_case1/ARE_First_Order_Derivative_[1,0,0]11 ==
  HDV_last_v : Inport
  Trigger : TriggerPort  TriggerType=either  VariantControl=Variant  ZeroCross=off  PortDimensions=1
  Constant : Constant  Value=T_ADE
  Constant52 : Constant  Value=HDV_last_v0
  MATLAB Function : MATLAB Function  TreatAsAtomicUnit=on
  HDV_last_v_dot_hat : Outport  VectorParamsAs1DForOutWhenUnconnected=off
  wires:
  Constant/1 -> MATLAB Function/2(Ts)
  MATLAB Function/1(Dot_U) -> HDV_last_v_dot_hat/1
  HDV_last_v/1 -> MATLAB Function/1(U)
  Constant52/1 -> MATLAB Function/3(u_init)

== system HDVPSG_DelayComp_NewRef_RealDrop_case1/ARE_First_Order_Derivative_[1,0,0]12 ==
  PSG_first_v : Inport
  Trigger : TriggerPort  TriggerType=either  VariantControl=Variant  ZeroCross=off  PortDimensions=1
  Constant : Constant  Value=T_ADE
  Constant52 : Constant  Value=PSG_first_v0
  MATLAB Function : MATLAB Function  TreatAsAtomicUnit=on
  PSG_first_v_dot_hat : Outport  VectorParamsAs1DForOutWhenUnconnected=off
  wires:
  Constant52/1 -> MATLAB Function/3(u_init)
  PSG_first_v/1 -> MATLAB Function/1(U)
  MATLAB Function/1(Dot_U) -> PSG_first_v_dot_hat/1
  Constant/1 -> MATLAB Function/2(Ts)

== system HDVPSG_DelayComp_NewRef_RealDrop_case1/ARE_First_Order_Derivative_[1,0,0]13 ==
  PSG_middle_v : Inport
  Trigger : TriggerPort  TriggerType=either  VariantControl=Variant  ZeroCross=off  PortDimensions=1
  Constant : Constant  Value=T_ADE
  Constant52 : Constant  Value=PSG_middle_v0
  MATLAB Function : MATLAB Function  TreatAsAtomicUnit=on
  PSG_middle_v_dot_hat : Outport  VectorParamsAs1DForOutWhenUnconnected=off
  wires:
  Constant/1 -> MATLAB Function/2(Ts)
  MATLAB Function/1(Dot_U) -> PSG_middle_v_dot_hat/1
  PSG_middle_v/1 -> MATLAB Function/1(U)
  Constant52/1 -> MATLAB Function/3(u_init)

== system HDVPSG_DelayComp_NewRef_RealDrop_case1/ARE_First_Order_Derivative_[1,0,0]14 ==
  HDV_first_v : Inport
  Trigger : TriggerPort  TriggerType=either  VariantControl=Variant  ZeroCross=off  PortDimensions=1
  Constant : Constant  Value=T_ADE
  Constant52 : Constant  Value=HDV_first_v0
  MATLAB Function : MATLAB Function  TreatAsAtomicUnit=on
  HDV_first_v_dot_hat : Outport  VectorParamsAs1DForOutWhenUnconnected=off
  wires:
  Constant52/1 -> MATLAB Function/3(u_init)
  HDV_first_v/1 -> MATLAB Function/1(U)
  MATLAB Function/1(Dot_U) -> HDV_first_v_dot_hat/1
  Constant/1 -> MATLAB Function/2(Ts)

== system HDVPSG_DelayComp_NewRef_RealDrop_case1/ARE_First_Order_Derivative_[1,0,0]15 ==
  PSG_end_v : Inport
  Trigger : TriggerPort  TriggerType=either  VariantControl=Variant  ZeroCross=off  PortDimensions=1
  Constant : Constant  Value=T_ADE
  Constant52 : Constant  Value=PSG_end_v0
  MATLAB Function : MATLAB Function  TreatAsAtomicUnit=on
  PSG_end_v_dot_hat : Outport  VectorParamsAs1DForOutWhenUnconnected=off
  wires:
  Constant52/1 -> MATLAB Function/3(u_init)
  PSG_end_v/1 -> MATLAB Function/1(U)
  MATLAB Function/1(Dot_U) -> PSG_end_v_dot_hat/1
  Constant/1 -> MATLAB Function/2(Ts)

== system HDVPSG_DelayComp_NewRef_RealDrop_case1/ARE_First_Order_Derivative_[1,0,0]2 ==
  PSG_first_v : Inport
  Trigger : TriggerPort  TriggerType=either  VariantControl=Variant  ZeroCross=off  PortDimensions=1
  Constant : Constant  Value=T_ADE
  Constant52 : Constant  Value=PSG_first_v0
  MATLAB Function : MATLAB Function  TreatAsAtomicUnit=on
  PSG_first_v_dot_hat : Outport  VectorParamsAs1DForOutWhenUnconnected=off
  wires:
  Constant/1 -> MATLAB Function/2(Ts)
  MATLAB Function/1(Dot_U) -> PSG_first_v_dot_hat/1
  PSG_first_v/1 -> MATLAB Function/1(U)
  Constant52/1 -> MATLAB Function/3(u_init)

== system HDVPSG_DelayComp_NewRef_RealDrop_case1/ARE_First_Order_Derivative_[1,0,0]3 ==
  HDV_First_v : Inport
  HDV_First_a : Inport  Port=2
  Enable : EnablePort
  HDV_First_v0_ctz : Outport  VectorParamsAs1DForOutWhenUnconnected=off
  HDV_First_a0_ctz : Outport  Port=2  VectorParamsAs1DForOutWhenUnconnected=off
  wires:
  HDV_First_v/1 -> HDV_First_v0_ctz/1
  HDV_First_a/1 -> HDV_First_a0_ctz/1

== system HDVPSG_DelayComp_NewRef_RealDrop_case1/ARE_First_Order_Derivative_[1,0,0]4 ==
  PSG_first_v : Inport
  Trigger : TriggerPort  TriggerType=either  VariantControl=Variant  ZeroCross=off  PortDimensions=1
  Constant : Constant  Value=T_ADE
  Constant52 : Constant  Value=PSG_first_v0
  MATLAB Function : MATLAB Function  TreatAsAtomicUnit=on
  PSG_first_v_dot_hat : Outport  VectorParamsAs1DForOutWhenUnconnected=off
  wires:
  Constant/1 -> MATLAB Function/2(Ts)
  MATLAB Function/1(Dot_U) -> PSG_first_v_dot_hat/1
  PSG_first_v/1 -> MATLAB Function/1(U)
  Constant52/1 -> MATLAB Function/3(u_init)

== system HDVPSG_DelayComp_NewRef_RealDrop_case1/ARE_First_Order_Derivative_[1,0,0]5 ==
  PSG_middle_v : Inport
  Trigger : TriggerPort  TriggerType=either  VariantControl=Variant  ZeroCross=off  PortDimensions=1
  Constant : Constant  Value=T_ADE
  Constant52 : Constant  Value=PSG_middle_v0
  MATLAB Function : MATLAB Function  TreatAsAtomicUnit=on
  PSG_middle_v_dot_hat : Outport  VectorParamsAs1DForOutWhenUnconnected=off
  wires:
  Constant52/1 -> MATLAB Function/3(u_init)
  PSG_middle_v/1 -> MATLAB Function/1(U)
  MATLAB Function/1(Dot_U) -> PSG_middle_v_dot_hat/1
  Constant/1 -> MATLAB Function/2(Ts)

== system HDVPSG_DelayComp_NewRef_RealDrop_case1/ARE_First_Order_Derivative_[1,0,0]6 ==
  HDV_First_v : Inport
  Trigger : TriggerPort  TriggerType=either  VariantControl=Variant  ZeroCross=off  PortDimensions=1
  Constant : Constant  Value=T_ADE
  Constant1 : Constant  Value=HDV_first_v0
  MATLAB Function : MATLAB Function  TreatAsAtomicUnit=on
  HDV_First_v_dot_hat : Outport  VectorParamsAs1DForOutWhenUnconnected=off
  wires:
  Constant1/1 -> MATLAB Function/3(u_init)
  HDV_First_v/1 -> MATLAB Function/1(U)
  MATLAB Function/1(Dot_U) -> HDV_First_v_dot_hat/1
  Constant/1 -> MATLAB Function/2(Ts)

== system HDVPSG_DelayComp_NewRef_RealDrop_case1/ARE_First_Order_Derivative_[1,0,0]7 ==
  HDV_last_v : Inport
  Trigger : TriggerPort  TriggerType=either  VariantControl=Variant  ZeroCross=off  PortDimensions=1
  Constant : Constant  Value=T_ADE
  Constant52 : Constant  Value=HDV_last_v0
  MATLAB Function : MATLAB Function  TreatAsAtomicUnit=on
  HDV_last_v_dot_hat : Outport  VectorParamsAs1DForOutWhenUnconnected=off
  wires:
  Constant52/1 -> MATLAB Function/3(u_init)
  HDV_last_v/1 -> MATLAB Function/1(U)
  MATLAB Function/1(Dot_U) -> HDV_last_v_dot_hat/1
  Constant/1 -> MATLAB Function/2(Ts)

== system HDVPSG_DelayComp_NewRef_RealDrop_case1/ARE_First_Order_Derivative_[1,0,0]8 ==
  PSG_middle_v : Inport
  Trigger : TriggerPort  TriggerType=either  VariantControl=Variant  ZeroCross=off  PortDimensions=1
  Constant : Constant  Value=T_ADE
  Constant52 : Constant  Value=PSG_middle_v0
  MATLAB Function : MATLAB Function  TreatAsAtomicUnit=on
  PSG_middle_v_dot_hat : Outport  VectorParamsAs1DForOutWhenUnconnected=off
  wires:
  Constant52/1 -> MATLAB Function/3(u_init)
  PSG_middle_v/1 -> MATLAB Function/1(U)
  MATLAB Function/1(Dot_U) -> PSG_middle_v_dot_hat/1
  Constant/1 -> MATLAB Function/2(Ts)

== system HDVPSG_DelayComp_NewRef_RealDrop_case1/ARE_First_Order_Derivative_[1,0,0]9 ==
  PSG_end_v : Inport
  Trigger : TriggerPort  TriggerType=either  VariantControl=Variant  ZeroCross=off  PortDimensions=1
  Constant : Constant  Value=T_ADE
  Constant52 : Constant  Value=PSG_end_v0
  MATLAB Function : MATLAB Function  TreatAsAtomicUnit=on
  PSG_end_v_dot_hat : Outport  VectorParamsAs1DForOutWhenUnconnected=off
  wires:
  Constant/1 -> MATLAB Function/2(Ts)
  MATLAB Function/1(Dot_U) -> PSG_end_v_dot_hat/1
  PSG_end_v/1 -> MATLAB Function/1(U)
  Constant52/1 -> MATLAB Function/3(u_init)
